simulink model "untitled"  (R2020b)
settings: Solver=VariableStepAuto  StartTime=0.0  StopTime=500  FixedStep=0.000001  MaxStep=1e-4  RelTol=1e-3  EnableMultiTasking=on
libraries: dsparch4 x5, dspsrcs4 x4, simulink x2, dspfdesign x2
(part 4 of 4)

== matlab function untitled/MATLAB Function ==
  data: u input; y output
function y = fcn(u)

y = 2 * sqrt(u);

== matlab function untitled/MATLAB Function1 ==
  data: u input; y output
function y = fcn(u)

y = 2 * sqrt(u);
